simulink model "scattering_pos_pos_simo"  (R2022b)
settings: Solver=VariableStepAuto  StartTime=0.0  StopTime=10.0  RelTol=1e-3
values from neighbouring files (symbols this model uses):
  A = 2    [scattering_params.m]    (also in scattering_params_force_pos.m = 3; scattering_params_pos_pos.m = 3)
  b = 1    [scattering_params.m]    (also in scattering_params_force_pos.m = 40; scattering_params_pos_pos.m = 100)
  Be = 100    [scattering_params.m]    (also in scattering_params_force_pos.m; scattering_params_pos_pos.m)
  Bh = 1.5    [scattering_params.m]    (also in scattering_params_force_pos.m = 1; scattering_params_pos_pos.m = 1)
  Dh = 0.1    [scattering_params.m]    (also in scattering_params_force_pos.m = 16; scattering_params_pos_pos.m = 16)
  discrete_delay = 100    [scattering_params_force_pos.m]    (also in scattering_params_pos_pos.m)
  Fc = 1    [scattering_params.m]    (also in scattering_params_force_pos.m = 0.25; scattering_params_pos_pos.m = 0.25)
  Flp = 5    [scattering_params.m]    (also in scattering_params_force_pos.m = 0.5; scattering_params_pos_pos.m = 0.5)
  Jh = 1    [scattering_params.m]    (also in scattering_params_force_pos.m; scattering_params_pos_pos.m)
  Ke = 200    [scattering_params.m]    (also in scattering_params_force_pos.m; scattering_params_pos_pos.m)
  Mm = 0.5    [scattering_params.m]    (also in scattering_params_force_pos.m; scattering_params_pos_pos.m)
  Ms = 2    [scattering_params.m]    (also in scattering_params_force_pos.m; scattering_params_pos_pos.m)
  Ph = 10    [scattering_params.m]    (also in scattering_params_force_pos.m; scattering_params_pos_pos.m)
  scattering_filter_freq = 10    [scattering_params.m]    (also in scattering_params_force_pos.m; scattering_params_pos_pos.m)
  Ts = 0.001    [scattering_params_force_pos.m]    (also in scattering_params_pos_pos.m)
  xe = 5    [scattering_params.m]    (also in scattering_params_force_pos.m = 2; scattering_params_pos_pos.m = 2)
settings Model: Creator=Manu  LastModifiedBy=Manu

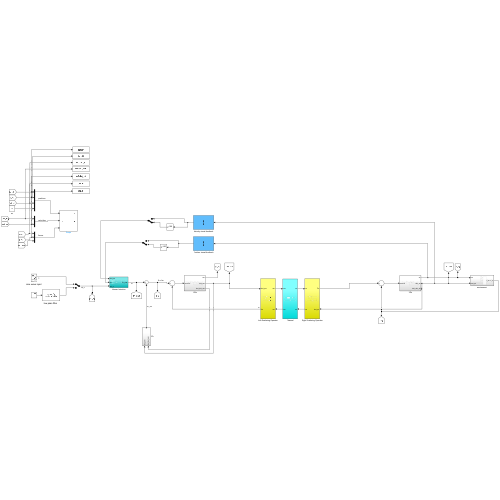
[thumbnail: Simulink's stored preview of the top-level diagram]
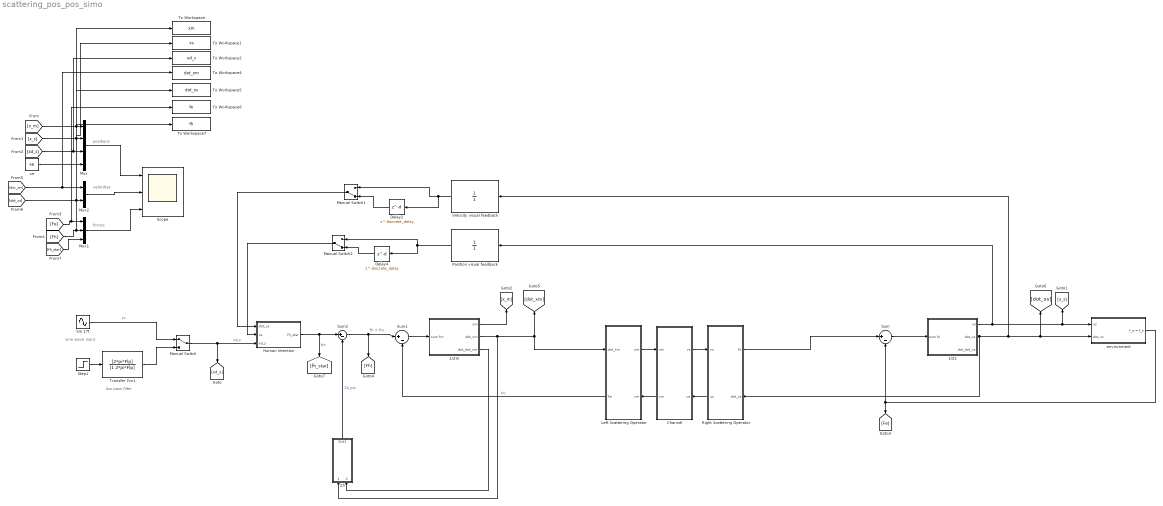
== system scattering_pos_pos_simo ==
  note: fh = fm
  note: sine wave input
  note: low pass filter
  note: positions
  note: forces
  note: velocities
  1/Zm : Subsystem
  1/Zs : Subsystem
  Channel : Subsystem
      settings: PortSchema="{\"entries\":[{\"content\":{\"sides\":[{\"content\":{\"connectorIds\":[\"In1\",\"Out2\"]},\"type\":\"ConnectorPlacement.EquallySpacedRectSide\",\"uuid\":\"b161512c-b7ed-4ebb-a20d-241659dc3c5a\"},{\"content\":{\"connectorIds\":[\"Out1\",\"In2\"],\"side\":\"RIGHT\"},\"type\":\"ConnectorPlacement.EquallySpacedRectSide\",\"uuid\":\"4974f610-b012-48cc-aa6a-5b8d68d9d4c6\"},{\"content\":{\"connectorIds\":[],\"side\":\"TOP\"},\"type\":\"ConnectorPlacement.EquallySpacedRectSide\",\"uuid\":\"82c908c3-5ed1-4ef0-8a50-6fa49874d665\"}]},\"type\":\"ConnectorPlacement.EquallySpacedConnector\",\"uuid\":\"454123fe-4b67-4aa7-9fc5-8cdd5b24b8fb\"}],\"packageUris\":[\"http://schema.mathworks.com/mf0/Connector/R2020b\"],\"version\":\"1.0\"}"
  Delay2 : Delay  DelayLength=discrete_delay  SampleTime=Ts
  Delay4 : Delay  DelayLength=discrete_delay  SampleTime=Ts
  Human Intention : Subsystem
  Left Scattering Operator : Subsystem
      settings: PortSchema="{\"entries\":[{\"content\":{\"sides\":[{\"content\":{\"connectorIds\":[\"In1\",\"Out2\"]},\"type\":\"ConnectorPlacement.EquallySpacedRectSide\",\"uuid\":\"b161512c-b7ed-4ebb-a20d-241659dc3c5a\"},{\"content\":{\"connectorIds\":[\"Out1\",\"In2\"],\"side\":\"RIGHT\"},\"type\":\"ConnectorPlacement.EquallySpacedRectSide\",\"uuid\":\"4974f610-b012-48cc-aa6a-5b8d68d9d4c6\"},{\"content\":{\"connectorIds\":[],\"side\":\"TOP\"},\"type\":\"ConnectorPlacement.EquallySpacedRectSide\",\"uuid\":\"82c908c3-5ed1-4ef0-8a50-6fa49874d665\"}]},\"type\":\"ConnectorPlacement.EquallySpacedConnector\",\"uuid\":\"454123fe-4b67-4aa7-9fc5-8cdd5b24b8fb\"}],\"packageUris\":[\"http://schema.mathworks.com/mf0/Connector/R2020b\"],\"version\":\"1.0\"}"
  Manual Switch : ManualSwitch
  Manual Switch1 : ManualSwitch  CurrentSetting=0
  Manual Switch2 : ManualSwitch  CurrentSetting=0
  Mux : Mux
  Mux1 : Mux  Inputs=3
  Mux2 : Mux  Inputs=2
  Position visual feedback : TransferFcn  Denominator=[1]
  Right Scattering Operator : Subsystem
      settings: PortSchema="{\"entries\":[{\"content\":{\"sides\":[{\"content\":{\"connectorIds\":[\"In1\",\"Out2\"]},\"type\":\"ConnectorPlacement.EquallySpacedRectSide\",\"uuid\":\"b161512c-b7ed-4ebb-a20d-241659dc3c5a\"},{\"content\":{\"connectorIds\":[\"Out1\",\"In2\"],\"side\":\"RIGHT\"},\"type\":\"ConnectorPlacement.EquallySpacedRectSide\",\"uuid\":\"4974f610-b012-48cc-aa6a-5b8d68d9d4c6\"},{\"content\":{\"connectorIds\":[],\"side\":\"TOP\"},\"type\":\"ConnectorPlacement.EquallySpacedRectSide\",\"uuid\":\"82c908c3-5ed1-4ef0-8a50-6fa49874d665\"}]},\"type\":\"ConnectorPlacement.EquallySpacedConnector\",\"uuid\":\"454123fe-4b67-4aa7-9fc5-8cdd5b24b8fb\"}],\"packageUris\":[\"http://schema.mathworks.com/mf0/Connector/R2020b\"],\"version\":\"1.0\"}"
  Scope : Scope  NumInputPorts=3
  Sin 17t : Sin  Amplitude=A  Frequency=2*pi*Fc  SampleTime=0
  Step1 : Step  Time=0.5  After=A  SampleTime=0
  Sum : Sum  Inputs=|+-
  Sum1 : Sum  Inputs=|+-
  Sum2 : Sum  Inputs=|+-
  To Workspace : ToWorkspace  VariableName=xm  SaveFormat=Timeseries  SampleTime=-1
  To Workspace1 : ToWorkspace  VariableName=xs  SaveFormat=Timeseries  SampleTime=-1
  To Workspace2 : ToWorkspace  VariableName=xd_s  SaveFormat=Timeseries  SampleTime=-1
  To Workspace4 : ToWorkspace  VariableName=dot_xm  SaveFormat=Timeseries  SampleTime=-1
  To Workspace5 : ToWorkspace  VariableName=dot_xs  SaveFormat=Timeseries  SampleTime=-1
  To Workspace6 : ToWorkspace  VariableName=fe  SaveFormat=Timeseries  SampleTime=-1
  To Workspace7 : ToWorkspace  VariableName=fh  SaveFormat=Timeseries  SampleTime=-1
  Transfer Fcn1 : TransferFcn  Numerator=[2*pi*Flp]  Denominator=[1 2*pi*Flp]
  Velocity visual feedback : TransferFcn  Denominator=[1]
  Zh : Subsystem
  environment : Subsystem
  xe : Constant  Value=xe
  wires:
  1/Zm/1(xm) -> [x_m]
  Manual Switch/1 -> [xd_s], Human Intention/3(xd_s)  "xd_s"
  Zh/1(Out1) -> Sum2/2  "Zh_out"
  Sin 17t/1 -> Manual Switch/1  "F*"
  1/Zm/3(dot_dot_xm) -> Zh/2(dot_dot_xm)
  Human Intention/1(fh_star) -> Sum2/1, [fh_star]  "fh*"
  Transfer Fcn1/1 -> Manual Switch/2
  Step1/1 -> Transfer Fcn1/1
  Sum2/1 -> [Fh], Sum1/1
  Sum1/1 -> 1/Zm/1(sum fm)
  Sum/1 -> 1/Zs/1(sum fs)
  1/Zs/2(dot_xs) -> Right Scattering Operator/2(dot_xs), Velocity visual feedback/1, [dot_xs], environment/2(dot_xs)
  1/Zs/1(xs) -> [x_s], environment/1(xs), Position visual feedback/1
  environment/1(f_e = f_s) -> [Fe], Sum/2
  Velocity visual feedback/1 -> Delay2/1, Manual Switch1/1
  Manual Switch1/1 -> Human Intention/1(dot_xs)
  Delay4/1 -> Manual Switch2/2
  Position visual feedback/1 -> Delay4/1, Manual Switch2/1
  Manual Switch2/1 -> Human Intention/2(xs)
  1/Zm/2(dot_xm) -> Left Scattering Operator/1(dot_xm), [dot_xm], Zh/1(dot_xm)
  Delay2/1 -> Manual Switch1/2
  [fh_star] -> Mux1/3
  Mux2/1 -> Scope/2
  [Fh] -> To Workspace7/1, Mux1/2
  [dot_xs] -> To Workspace5/1, Mux2/2
  [dot_xm] -> Mux2/1, To Workspace4/1
  [x_s] -> To Workspace1/1, Mux/2
  [x_m] -> To Workspace/1, Mux/1
  Mux1/1 -> Scope/3
  Mux/1 -> Scope/1
  xe/1 -> Mux/4
  [Fe] -> Mux1/1, To Workspace6/1
  [xd_s] -> To Workspace2/1, Mux/3
  Channel/2(vm) -> Left Scattering Operator/2(vm)
  Right Scattering Operator/2(us) -> Channel/2(us)
  Left Scattering Operator/1(um) -> Channel/1(um)
  Channel/1(vs) -> Right Scattering Operator/1(vs)
  Right Scattering Operator/1(Fs) -> Sum/1
  Left Scattering Operator/2(fm) -> Sum1/2  "fm"

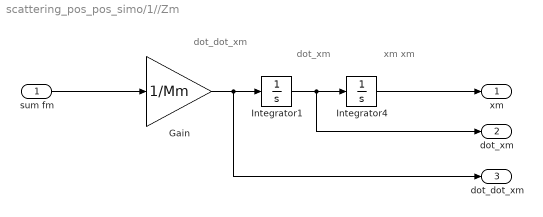
== system scattering_pos_pos_simo/1//Zm ==
  note: dot_dot_xm
  note: dot_xm
  note: xm
      | xm
  sum fm : Inport
  Gain : Gain  Gain=1/Mm
  Integrator1 : Integrator
  Integrator4 : Integrator
  xm : Outport
  dot_xm : Outport  Port=2
  dot_dot_xm : Outport  Port=3
  wires:
  sum fm/1 -> Gain/1
  Gain/1 -> dot_dot_xm/1, Integrator1/1
  Integrator4/1 -> xm/1
  Integrator1/1 -> dot_xm/1, Integrator4/1

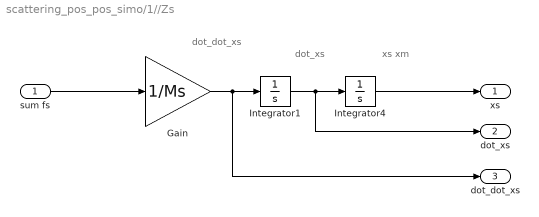
== system scattering_pos_pos_simo/1//Zs ==
  note: dot_dot_xs
  note: dot_xs
  note: xs
      | xm
  sum fs : Inport
  Gain : Gain  Gain=1/Ms
  Integrator1 : Integrator
  Integrator4 : Integrator
  xs : Outport
  dot_xs : Outport  Port=2
  dot_dot_xs : Outport  Port=3
  wires:
  sum fs/1 -> Gain/1
  Gain/1 -> dot_dot_xs/1, Integrator1/1
  Integrator4/1 -> xs/1
  Integrator1/1 -> dot_xs/1, Integrator4/1

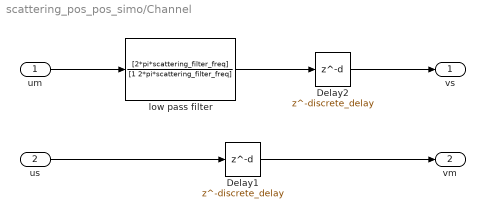
== system scattering_pos_pos_simo/Channel ==
  um : Inport
  us : Inport  Port=2
  Delay1 : Delay  DelayLength=discrete_delay  SampleTime=Ts
  Delay2 : Delay  DelayLength=discrete_delay  SampleTime=Ts
  low pass filter : TransferFcn  Numerator=[2*pi*scattering_filter_freq]  Denominator=[1 2*pi*scattering_filter_freq]
  vs : Outport
  vm : Outport  Port=2
  wires:
  um/1 -> low pass filter/1
  us/1 -> Delay1/1
  Delay1/1 -> vm/1
  Delay2/1 -> vs/1
  low pass filter/1 -> Delay2/1

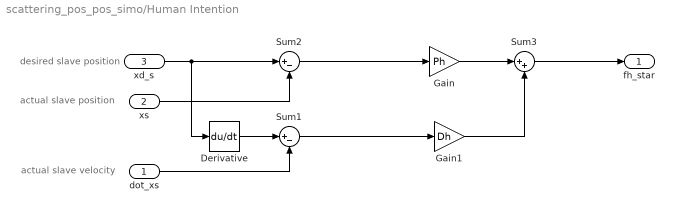
== system scattering_pos_pos_simo/Human Intention ==
  note: actual slave velocity
  note: actual slave position
  note: desired slave position
  dot_xs : Inport
  xs : Inport  Port=2
  xd_s : Inport  Port=3
  Derivative : Derivative
  Gain : Gain  Gain=Ph
  Gain1 : Gain  Gain=Dh
  Sum1 : Sum  Inputs=|+-
  Sum2 : Sum  Inputs=|+-
  Sum3 : Sum  Inputs=|++
  fh_star : Outport
  wires:
  xs/1 -> Sum2/2
  dot_xs/1 -> Sum1/2
  Sum2/1 -> Gain/1
  Sum1/1 -> Gain1/1
  Gain1/1 -> Sum3/2
  Gain/1 -> Sum3/1
  Sum3/1 -> fh_star/1
  xd_s/1 -> Derivative/1, Sum2/1
  Derivative/1 -> Sum1/1

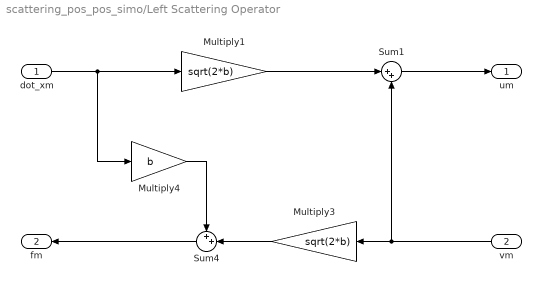
== system scattering_pos_pos_simo/Left Scattering Operator ==
  dot_xm : Inport
  vm : Inport  Port=2
  Multiply1 : Gain  Gain=sqrt(2*b)
  Multiply3 : Gain  Gain=sqrt(2*b)
  Multiply4 : Gain  Gain=b
  Sum1 : Sum  Inputs=|++
  Sum4 : Sum  Inputs=++|
  um : Outport
  fm : Outport  Port=2
  wires:
  Multiply1/1 -> Sum1/1
  Sum1/1 -> um/1
  dot_xm/1 -> Multiply4/1, Multiply1/1
  vm/1 -> Multiply3/1, Sum1/2
  Sum4/1 -> fm/1
  Multiply3/1 -> Sum4/2
  Multiply4/1 -> Sum4/1

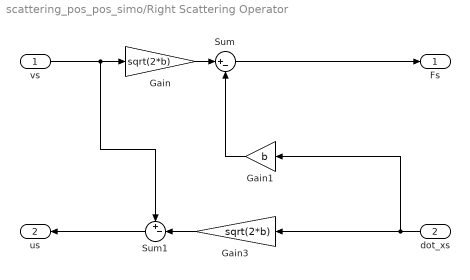
== system scattering_pos_pos_simo/Right Scattering Operator ==
  vs : Inport
  dot_xs : Inport  Port=2
  Gain : Gain  Gain=sqrt(2*b)
  Gain1 : Gain  Gain=b
  Gain3 : Gain  Gain=sqrt(2*b)
  Sum : Sum  Inputs=|+-
  Sum1 : Sum  Inputs=+-|
  Fs : Outport
  us : Outport  Port=2
  wires:
  dot_xs/1 -> Gain3/1, Gain1/1
  vs/1 -> Sum1/1, Gain/1
  Gain/1 -> Sum/1
  Sum/1 -> Fs/1
  Gain1/1 -> Sum/2
  Gain3/1 -> Sum1/2
  Sum1/1 -> us/1

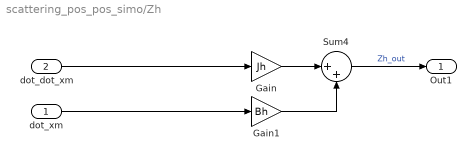
== system scattering_pos_pos_simo/Zh ==
  dot_xm : Inport
  dot_dot_xm : Inport  Port=2
  Gain : Gain  Gain=Jh
  Gain1 : Gain  Gain=Bh
  Sum4 : Sum  Inputs=|++
  Out1 : Outport
  wires:
  dot_dot_xm/1 -> Gain/1
  Gain1/1 -> Sum4/2
  Gain/1 -> Sum4/1
  Sum4/1 -> Out1/1  "Zh_out"
  dot_xm/1 -> Gain1/1

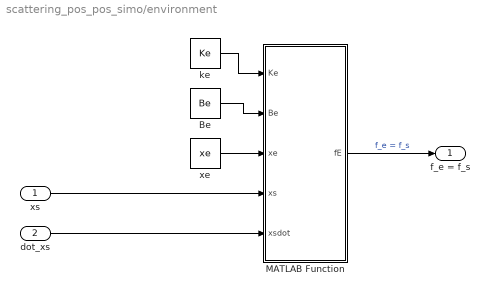
== system scattering_pos_pos_simo/environment ==
  xs : Inport
  dot_xs : Inport  Port=2
  Be : Constant  Value=Be
  MATLAB Function : MATLAB Function  TreatAsAtomicUnit=on
  ke : Constant  Value=Ke
  xe : Constant  Value=xe
  f_e = f_s : Outport
  wires:
  MATLAB Function/1(fE) -> f_e = f_s/1  "f_e = f_s"
  xs/1 -> MATLAB Function/4(xs)
  xe/1 -> MATLAB Function/3(xe)
  dot_xs/1 -> MATLAB Function/5(xsdot)
  ke/1 -> MATLAB Function/1(Ke)
  Be/1 -> MATLAB Function/2(Be)

== matlab function scattering_pos_pos_simo/environment/MATLAB Function ==
  data: Ke input; fE output; Be input; xe input; xs input; xsdot input
function fE = environment(Ke, Be, xe, xs, xsdot)
    if xs > xe
        fE = Ke * (xs - xe) + Be * xsdot; % Plot both contributions Ke and Be
    else
        fE = 0;
    end
end
